simulink model "SOCPIControlBenchmarkRealVarLParGH"  (R2019b)
settings: Solver=FixedStepAuto  StartTime=0.0  StopTime=50000  FixedStep=0.01  RelTol=1e-3
values from neighbouring files (symbols this model uses):
  kio = 0.6    [benchmarkPIDStartRealVarLParGH.m]
  kpo = 0.11    [benchmarkPIDStartRealVarLParGH.m]
  maxKi = 0.3    [benchmarkPIDStartRealVarLParGH.m]
  maxKp = 0.3    [benchmarkPIDStartRealVarLParGH.m]
  minKi = 0.01    [benchmarkPIDStartRealVarLParGH.m]
  minKp = 0.01    [benchmarkPIDStartRealVarLParGH.m]
  N = 100    [benchmarkPIDStartRealVarLParGH.m]
  optimPeriod = 300    [benchmarkPIDStartRealVarLParGH.m]
  OVLim = 5    [benchmarkPIDStartRealVarLParGH.m]
  refAmplitude = 50    [benchmarkPIDStartRealVarLParGH.m]
  refSignalPeriod = optimPeriod    (= 300)    [benchmarkPIDStartRealVarLParGH.m]
  resetThreshold = 0.1    [benchmarkPIDStartRealVarLParGH.m]
undefined symbols (not defined in the file or in its folder): sigbuilder_block
libraries: dspmathops x3, simulink x3
(part 1 of 2)
settings Model: Creator=jairo  LastModifiedBy=jairo
settings DataIOCC: ReturnWorkspaceOutputs=off

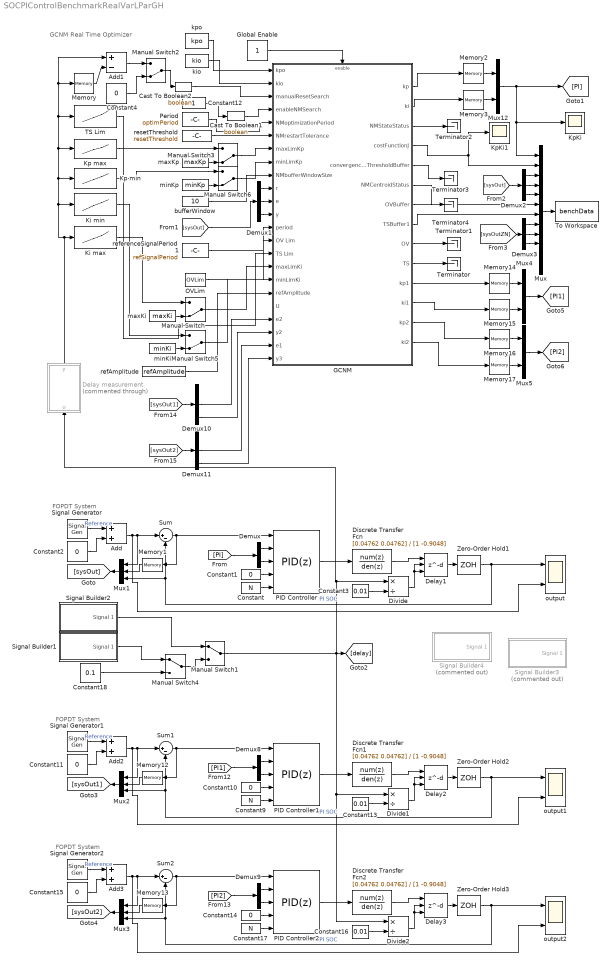
== system SOCPIControlBenchmarkRealVarLParGH ==
  note: FOPDT System
  note: GCNM Real Time Optimizer
  note: FOPDT System
  note: FOPDT System
  Add : Sum
  Add1 : Sum  Inputs=+-
  Add2 : Sum
  Add3 : Sum
  Cast To Boolean1 : DataTypeConversion  OutDataTypeStr=boolean
  Cast To Boolean2 : DataTypeConversion  OutDataTypeStr=boolean
  Constant : Constant  Value=N
  Constant{1..2,4,10..11,14..15} (7 alike) : Constant  Value=0
  Constant12 : Constant  OutDataTypeStr=boolean
  Constant13 : Constant  Value=0.01
  Constant16 : Constant  Value=0.01
  Constant17 : Constant  Value=N
  Constant18 : Constant  Value=0.1
  Constant3 : Constant  Value=0.01
  Constant9 : Constant  Value=N
  Delay measurement : MATLAB Function  Commented=through  TreatAsAtomicUnit=on
  Delay1 : Delay  DelayLengthSource=Input port  DelayLengthUpperLimit=1000  InitialConditionSource=Input port
      settings: InputPortMap=u0,p1,p4
  Delay2 : Delay  DelayLengthSource=Input port  DelayLengthUpperLimit=1000  InitialConditionSource=Input port
      settings: InputPortMap=u0,p1,p4
  Delay3 : Delay  DelayLengthSource=Input port  DelayLengthUpperLimit=1000  InitialConditionSource=Input port
      settings: InputPortMap=u0,p1,p4
  Demux : Demux  Outputs=2
  Demux{1..3,10..11} (5 alike) : Demux  Outputs=3
  Demux8 : Demux  Outputs=2
  Demux9 : Demux  Outputs=2
  Discrete Transfer Fcn : DiscreteTransferFcn  Numerator=[0.04762 0.04762]  Denominator=[1 -0.9048]
  Discrete Transfer Fcn1 : DiscreteTransferFcn  Numerator=[0.04762 0.04762]  Denominator=[1 -0.9048]
  Discrete Transfer Fcn2 : DiscreteTransferFcn  Numerator=[0.04762 0.04762]  Denominator=[1 -0.9048]
  Divide : Product  Inputs=*/
  Divide1 : Product  Inputs=*/
  Divide2 : Product  Inputs=*/
  GCNM : Subsystem
  Global Enable : Constant
  Ki max : Lookup_n-D  NumberOfTableDimensions=1  BreakpointsForDimension1=[0.1 0.5 1 2 3 4 5 6 7 8 9 10]  UseOneInputPortForAllInputData=on  Table=|  InternalRulePriority=Speed  RndMeth=Simplest  InputSameDT=on
      | [3
      | 1.61
      | 0.9
      | 0.4
      | 0.4
      | 0.3
      | 0.18
      | 0.15
      | 0.12
      | 0.1
      | 0.09
      | 0.07]
  Ki min : Lookup_n-D  NumberOfTableDimensions=1  BreakpointsForDimension1=[0.1 0.5 1 2 3 4 5 6 7 8 9 10]  UseOneInputPortForAllInputData=on  Table=|  InternalRulePriority=Speed  RndMeth=Simplest  InputSameDT=on
      | [0.8
      | 0.41
      | 0.21
      | 0.21
      | 0.11
      | 0.11
      | 0.061
      | 0.06
      | 0.061
      | 0.061
      | 0.061
      | 0.041]
  Kp max : Lookup_n-D  NumberOfTableDimensions=1  BreakpointsForDimension1=[0.1 0.5 1 2 3 4 5 6 7 8 9 10]  UseOneInputPortForAllInputData=on  Table=|  InternalRulePriority=Speed  RndMeth=Simplest  InputSameDT=on
      | [3
      | 2.21
      | 1.8
      | 1.1
      | 1
      | 0.9
      | 0.68
      | 0.73
      | 0.69
      | 0.67
      | 0.63
      | 0.54]
  Kp min : Lookup_n-D  NumberOfTableDimensions=1  BreakpointsForDimension1=[0.1 0.5 1 2 3 4 5 6 7 8 9 10]  UseOneInputPortForAllInputData=on  Table=|  InternalRulePriority=Speed  RndMeth=Simplest  InputSameDT=on
      | [0.1
      | 0.01
      | 0.01
      | 0.01
      | 0.01
      | 0.01
      | 0.01
      | 0.01
      | 0.01
      | 0.01
      | 0.01
      | 0.01
      | ]
  KpKi : Scope
  KpKi1 : Scope
  Manual Switch{,2..3,5..6} (5 alike) : ManualSwitch  CurrentSetting=0
  Manual Switch1 : ManualSwitch
  Manual Switch4 : ManualSwitch
  Memory{,1,12..13} (4 alike) : Memory
  Memory{14..17} (4 alike) : Memory  InitialCondition=0.1
  Memory2 : Memory  InitialCondition=kpo
  Memory3 : Memory  InitialCondition=kio
  Mux : Mux  Inputs=12
  Mux1 : Mux  Inputs=3
  Mux12 : Mux  Inputs=2
  Mux2 : Mux  Inputs=3
  Mux3 : Mux  Inputs=3
  Mux4 : Mux  Inputs=2
  Mux5 : Mux  Inputs=2
  OVLim : Constant  Value=OVLim
  PID Controller : simulink/Continuous/PID Controller  Controller=PID  Form=Parallel  TimeDomain=Discrete-time  SampleTime=0.1  IntegratorMethod=Forward Euler  FilterMethod=Forward Euler  ControllerParametersSource=external  P=1  I=100  D=0  UseFilter=on  N=100  TunerSelectOption=Transfer Function Based (PID Tuner App)  InitialConditionSource=internal  InitialConditionForIntegrator=0  InitialConditionForFilter=0  DifferentiatorICPrevScaledInput=0  ExternalReset=none  TrackingMode=off  Kt=1  LimitOutput=off  UpperSaturationLimit=inf  LowerSaturationLimit=-inf  LinearizeAsGain=on  AntiWindupMode=none  Kb=1  POutMin=[]  POutMax=[]  IOutMin=[]  IOutMax=[]  DOutMin=[]  DOutMax=[]  NOutMin=[]  NOutMax=[]  SumOutMin=[]  SumOutMax=[]  SaturationOutMin=[]  SaturationOutMax=[]  PParamMin=[]  PParamMax=[]  IParamMin=[]  IParamMax=[]  DParamMin=[]  DParamMax=[]  NParamMin=[]  NParamMax=[]  KbParamMin=[]  KbParamMax=[]  KtParamMin=[]  KtParamMax=[]  KbOutMin=[]  KbOutMax=[]  KtOutMin=[]  KtOutMax=[]  IntegratorOutMin=[]  IntegratorOutMax=[]  FilterOutMin=[]  FilterOutMax=[]  SumI1OutMin=[]  SumI1OutMax=[]  SumI2OutMin=[]  SumI2OutMax=[]  SumI3OutMin=[]  SumI3OutMax=[]  SumI4OutMin=[]  SumI4OutMax=[]  SumDOutMin=[]  SumDOutMax=[]  DifferentiatorOutMin=[]  DifferentiatorOutMax=[]  FilterDiffOutCoefMin=[]  FilterDiffOutCoefMax=[]  ReciprocalOutMin=[]  ReciprocalOutMax=[]  SumDenOutMin=[]  SumDenOutMax=[]  SumNumOutMin=[]  SumNumOutMax=[]  DivideOutMin=[]  DivideOutMax=[]  IntegratorContinuousStateAttributes=''  IntegratorStateMustResolveToSignalObject=off  IntegratorRTWStateStorageClass=Auto  FilterContinuousStateAttributes=''  FilterStateMustResolveToSignalObject=off  FilterRTWStateStorageClass=Auto  ParallelPVariant=ExternalParameters  IdealPVariant=Disabled  IVariant=ExternalParameters  DVariant=ExternalParameters  IntegratorVariant=Discrete  SatVariant=Disabled  AWVariant=Passthrough  PCopyVariant=Disabled  TRVariant=Disabled  FdbkBlocksVariant=Forward  IdealPFdbkVariant=Disabled  SatFdbkVariant=Disabled  DerivativeFilterVariant=ForwardEulerFilter  NVariant=ExternalParameters  NCopyVariant=Disabled  FilterICVariant=InternalICsFilter  IntegratorICVariant=InternalICs  ExternalResetVariant=Disabled  TRSumVariant=Passthrough  SumFdbkVariant=Disabled  SumVariant=Sum_PID
  PID Controller1 : simulink/Continuous/PID Controller  Controller=PID  Form=Parallel  TimeDomain=Discrete-time  SampleTime=0.1  IntegratorMethod=Forward Euler  FilterMethod=Forward Euler  ControllerParametersSource=external  P=1  I=100  D=0  UseFilter=on  N=100  TunerSelectOption=Transfer Function Based (PID Tuner App)  InitialConditionSource=internal  InitialConditionForIntegrator=0  InitialConditionForFilter=0  DifferentiatorICPrevScaledInput=0  ExternalReset=none  TrackingMode=off  Kt=1  LimitOutput=off  UpperSaturationLimit=inf  LowerSaturationLimit=-inf  LinearizeAsGain=on  AntiWindupMode=none  Kb=1  POutMin=[]  POutMax=[]  IOutMin=[]  IOutMax=[]  DOutMin=[]  DOutMax=[]  NOutMin=[]  NOutMax=[]  SumOutMin=[]  SumOutMax=[]  SaturationOutMin=[]  SaturationOutMax=[]  PParamMin=[]  PParamMax=[]  IParamMin=[]  IParamMax=[]  DParamMin=[]  DParamMax=[]  NParamMin=[]  NParamMax=[]  KbParamMin=[]  KbParamMax=[]  KtParamMin=[]  KtParamMax=[]  KbOutMin=[]  KbOutMax=[]  KtOutMin=[]  KtOutMax=[]  IntegratorOutMin=[]  IntegratorOutMax=[]  FilterOutMin=[]  FilterOutMax=[]  SumI1OutMin=[]  SumI1OutMax=[]  SumI2OutMin=[]  SumI2OutMax=[]  SumI3OutMin=[]  SumI3OutMax=[]  SumI4OutMin=[]  SumI4OutMax=[]  SumDOutMin=[]  SumDOutMax=[]  DifferentiatorOutMin=[]  DifferentiatorOutMax=[]  FilterDiffOutCoefMin=[]  FilterDiffOutCoefMax=[]  ReciprocalOutMin=[]  ReciprocalOutMax=[]  SumDenOutMin=[]  SumDenOutMax=[]  SumNumOutMin=[]  SumNumOutMax=[]  DivideOutMin=[]  DivideOutMax=[]  IntegratorContinuousStateAttributes=''  IntegratorStateMustResolveToSignalObject=off  IntegratorRTWStateStorageClass=Auto  FilterContinuousStateAttributes=''  FilterStateMustResolveToSignalObject=off  FilterRTWStateStorageClass=Auto  ParallelPVariant=ExternalParameters  IdealPVariant=Disabled  IVariant=ExternalParameters  DVariant=ExternalParameters  IntegratorVariant=Discrete  SatVariant=Disabled  AWVariant=Passthrough  PCopyVariant=Disabled  TRVariant=Disabled  FdbkBlocksVariant=Forward  IdealPFdbkVariant=Disabled  SatFdbkVariant=Disabled  DerivativeFilterVariant=ForwardEulerFilter  NVariant=ExternalParameters  NCopyVariant=Disabled  FilterICVariant=InternalICsFilter  IntegratorICVariant=InternalICs  ExternalResetVariant=Disabled  TRSumVariant=Passthrough  SumFdbkVariant=Disabled  SumVariant=Sum_PID
  PID Controller2 : simulink/Continuous/PID Controller  Controller=PID  Form=Parallel  TimeDomain=Discrete-time  SampleTime=0.1  IntegratorMethod=Forward Euler  FilterMethod=Forward Euler  ControllerParametersSource=external  P=1  I=100  D=0  UseFilter=on  N=100  TunerSelectOption=Transfer Function Based (PID Tuner App)  InitialConditionSource=internal  InitialConditionForIntegrator=0  InitialConditionForFilter=0  DifferentiatorICPrevScaledInput=0  ExternalReset=none  TrackingMode=off  Kt=1  LimitOutput=off  UpperSaturationLimit=inf  LowerSaturationLimit=-inf  LinearizeAsGain=on  AntiWindupMode=none  Kb=1  POutMin=[]  POutMax=[]  IOutMin=[]  IOutMax=[]  DOutMin=[]  DOutMax=[]  NOutMin=[]  NOutMax=[]  SumOutMin=[]  SumOutMax=[]  SaturationOutMin=[]  SaturationOutMax=[]  PParamMin=[]  PParamMax=[]  IParamMin=[]  IParamMax=[]  DParamMin=[]  DParamMax=[]  NParamMin=[]  NParamMax=[]  KbParamMin=[]  KbParamMax=[]  KtParamMin=[]  KtParamMax=[]  KbOutMin=[]  KbOutMax=[]  KtOutMin=[]  KtOutMax=[]  IntegratorOutMin=[]  IntegratorOutMax=[]  FilterOutMin=[]  FilterOutMax=[]  SumI1OutMin=[]  SumI1OutMax=[]  SumI2OutMin=[]  SumI2OutMax=[]  SumI3OutMin=[]  SumI3OutMax=[]  SumI4OutMin=[]  SumI4OutMax=[]  SumDOutMin=[]  SumDOutMax=[]  DifferentiatorOutMin=[]  DifferentiatorOutMax=[]  FilterDiffOutCoefMin=[]  FilterDiffOutCoefMax=[]  ReciprocalOutMin=[]  ReciprocalOutMax=[]  SumDenOutMin=[]  SumDenOutMax=[]  SumNumOutMin=[]  SumNumOutMax=[]  DivideOutMin=[]  DivideOutMax=[]  IntegratorContinuousStateAttributes=''  IntegratorStateMustResolveToSignalObject=off  IntegratorRTWStateStorageClass=Auto  FilterContinuousStateAttributes=''  FilterStateMustResolveToSignalObject=off  FilterRTWStateStorageClass=Auto  ParallelPVariant=ExternalParameters  IdealPVariant=Disabled  IVariant=ExternalParameters  DVariant=ExternalParameters  IntegratorVariant=Discrete  SatVariant=Disabled  AWVariant=Passthrough  PCopyVariant=Disabled  TRVariant=Disabled  FdbkBlocksVariant=Forward  IdealPFdbkVariant=Disabled  SatFdbkVariant=Disabled  DerivativeFilterVariant=ForwardEulerFilter  NVariant=ExternalParameters  NCopyVariant=Disabled  FilterICVariant=InternalICsFilter  IntegratorICVariant=InternalICs  ExternalResetVariant=Disabled  TRSumVariant=Passthrough  SumFdbkVariant=Disabled  SumVariant=Sum_PID
  Period : Constant  Value=optimPeriod  OutDataTypeStr=double
  Signal Generator : SignalGenerator  WaveForm=square  Frequency=1/refSignalPeriod
  Signal Generator1 : SignalGenerator  WaveForm=square  Frequency=1/refSignalPeriod
  Signal Generator2 : SignalGenerator  WaveForm=square  Frequency=1/refSignalPeriod
  Signal Builder1 : Subsystem  Tag=STV Subsys  LoadFcn=sigbuilder_block('load');  StartFcn=sigbuilder_block('start');  StopFcn=sigbuilder_block('stop');  ClipboardFcn=sigbuilder_block('clipboard');  mask(Sigbuilder block){tuvar=[0:10]}
      mask help: Simulink:masks:SigbuilderBlock_MD
      mask init:
      | if ~strcmp(get_param(bdroot(gcbh),'SimulationStatus'),'stopped') tuvar = sigbuilder_block('maskInit'); end
      settings: CopyFcn=sigbuilder_block('copy');  DeleteFcn=sigbuilder_block('delete');  ModelCloseFcn=sigbuilder_block('modelClose');  PreSaveFcn=sigbuilder_block('preSave');  PauseFcn=sigbuilder_block('pause');  ContinueFcn=sigbuilder_block('continue');  NameChangeFcn=sigbuilder_block('namechange');  OpenFcn=sigbuilder_block('open',[5.4 30.6 1141.2 522.6 ]);  CloseFcn=sigbuilder_block('close');
      mask Display: plot(0, 0, 100, 100,[2, 2, 32, 32, 2], [68, 8, 8, 68, 68],[32, 2], [38, 38], [32, 19, 2],[53, 60, 44], [32, 17, 17, 2],[16, 16, 31, 31]);txt = getActiveGroup(gcbh);text(2, 100, txt,'verticalAlignment', 'top');
  Signal Builder2 : Subsystem  Tag=STV Subsys  LoadFcn=sigbuilder_block('load',[0.75 38.25 1141.5 514.5 ]);  StartFcn=sigbuilder_block('start');  StopFcn=sigbuilder_block('stop');  ClipboardFcn=sigbuilder_block('clipboard');  mask(Sigbuilder block){tuvar=[0:10]}
      mask help: Simulink:masks:SigbuilderBlock_MD
      mask init:
      | if ~strcmp(get_param(bdroot(gcbh),'SimulationStatus'),'stopped') tuvar = sigbuilder_block('maskInit'); end
      settings: CopyFcn=sigbuilder_block('copy');  DeleteFcn=sigbuilder_block('delete');  ModelCloseFcn=sigbuilder_block('modelClose');  PreSaveFcn=sigbuilder_block('preSave');  PauseFcn=sigbuilder_block('pause');  ContinueFcn=sigbuilder_block('continue');  NameChangeFcn=sigbuilder_block('namechange');  OpenFcn=sigbuilder_block('open',[0.75 38.25 1141.5 514.5 ]);  CloseFcn=sigbuilder_block('close');
      mask Display: plot(0, 0, 100, 100,[2, 2, 32, 32, 2], [68, 8, 8, 68, 68],[32, 2], [38, 38], [32, 19, 2],[53, 60, 44], [32, 17, 17, 2],[16, 16, 31, 31]);txt = getActiveGroup(gcbh);text(2, 100, txt,'verticalAlignment', 'top');
  Signal Builder3 : Subsystem  Tag=STV Subsys  Commented=on  LoadFcn=sigbuilder_block('load');  StartFcn=sigbuilder_block('start');  StopFcn=sigbuilder_block('stop');  ClipboardFcn=sigbuilder_block('clipboard');  mask(Sigbuilder block){tuvar=[0:10]}
      mask help: Simulink:masks:SigbuilderBlock_MD
      mask init:
      | if ~strcmp(get_param(bdroot(gcbh),'SimulationStatus'),'stopped') tuvar = sigbuilder_block('maskInit'); end
      settings: CopyFcn=sigbuilder_block('copy');  DeleteFcn=sigbuilder_block('delete');  ModelCloseFcn=sigbuilder_block('modelClose');  PreSaveFcn=sigbuilder_block('preSave');  PauseFcn=sigbuilder_block('pause');  ContinueFcn=sigbuilder_block('continue');  NameChangeFcn=sigbuilder_block('namechange');  OpenFcn=sigbuilder_block('open',[5.4 33 1141.2 514.8 ]);  CloseFcn=sigbuilder_block('close');
      mask Display: plot(0, 0, 100, 100,[2, 2, 32, 32, 2], [68, 8, 8, 68, 68],[32, 2], [38, 38], [32, 19, 2],[53, 60, 44], [32, 17, 17, 2],[16, 16, 31, 31]);txt = getActiveGroup(gcbh);text(2, 100, txt,'verticalAlignment', 'top');
  Signal Builder4 : Subsystem  Tag=STV Subsys  Commented=on  LoadFcn=sigbuilder_block('load');  StartFcn=sigbuilder_block('start');  StopFcn=sigbuilder_block('stop');  ClipboardFcn=sigbuilder_block('clipboard');  mask(Sigbuilder block){tuvar=[0:10]}
      mask help: Simulink:masks:SigbuilderBlock_MD
      mask init:
      | if ~strcmp(get_param(bdroot(gcbh),'SimulationStatus'),'stopped') tuvar = sigbuilder_block('maskInit'); end
      settings: CopyFcn=sigbuilder_block('copy');  DeleteFcn=sigbuilder_block('delete');  ModelCloseFcn=sigbuilder_block('modelClose');  PreSaveFcn=sigbuilder_block('preSave');  PauseFcn=sigbuilder_block('pause');  ContinueFcn=sigbuilder_block('continue');  NameChangeFcn=sigbuilder_block('namechange');  OpenFcn=sigbuilder_block('open',[5.4 30.6 1141.2 522.6 ]);  CloseFcn=sigbuilder_block('close');
      mask Display: plot(0, 0, 100, 100,[2, 2, 32, 32, 2], [68, 8, 8, 68, 68],[32, 2], [38, 38], [32, 19, 2],[53, 60, 44], [32, 17, 17, 2],[16, 16, 31, 31]);txt = getActiveGroup(gcbh);text(2, 100, txt,'verticalAlignment', 'top');
  Sum : Sum  Inputs=|+-
  Sum1 : Sum  Inputs=|+-
  Sum2 : Sum  Inputs=|+-
  TS Lim : Lookup_n-D  NumberOfTableDimensions=1  BreakpointsForDimension1=[0.1 0.5 1 2 3 4 5 6 7 8 9 10]  UseOneInputPortForAllInputData=on  Table=|  InternalRulePriority=Speed  RndMeth=Simplest  InputSameDT=on
      | [100
      | 100
      | 100
      | 100
      | 100
      | 100
      | 100
      | 100
      | 100
      | 100
      | 100
      | 100]
  Terminator{,1..4} (5 alike) : Terminator
  To Workspace : ToWorkspace  VariableName=benchData  SaveFormat=Timeseries  SampleTime=-1
  Zero-Order Hold1 : ZeroOrderHold  SampleTime=-1
  Zero-Order Hold2 : ZeroOrderHold  SampleTime=-1
  Zero-Order Hold3 : ZeroOrderHold  SampleTime=-1
  bufferWindow : Constant  Value=10  OutDataTypeStr=uint16
  kio : Constant  Value=kio  OutDataTypeStr=double
  kpo : Constant  Value=kpo  OutDataTypeStr=double
  maxKi : Constant  Value=maxKi  VectorParams1D=off  OutDataTypeStr=double
  maxKp : Constant  Value=maxKp  OutDataTypeStr=double
  minKi : Constant  Value=minKi  OutDataTypeStr=double
  minKp : Constant  Value=minKp  OutDataTypeStr=double
  output : Scope  NumInputPorts=2
  output1 : Scope  NumInputPorts=2
  output2 : Scope  NumInputPorts=2
  refAmplitude : Constant  Value=refAmplitude  OutDataTypeStr=double
  referenceSignalPeriod1 : Constant  Value=refSignalPeriod
  resetThreshold : Constant  Value=resetThreshold
  wires:
  PID Controller/1 -> Discrete Transfer Fcn/1
  Sum/1 -> Memory1/1, PID Controller/1
  resetThreshold/1 -> GCNM/6(NMrestartTolerance)
  bufferWindow/1 -> GCNM/9(NMbufferWindowSize)
  Cast To Boolean1/1 -> GCNM/4(enableNMSearch)
  kio/1 -> GCNM/2(kio)
  Constant12/1 -> Cast To Boolean1/1
  Global Enable/1 -> GCNM/Enable
  kpo/1 -> GCNM/1(kpo)
  Period/1 -> GCNM/5(NMoptimizationPeriod)
  GCNM/4(costFunctionJ) -> Mux/2, KpKi1/1
  OVLim/1 -> GCNM/14("  OV Lim")
  Zero-Order Hold1/1 -> Sum/2, Mux1/3, output/1  "PI SOC"
  GCNM/1("  kp") -> Memory2/1
  GCNM/2("  ki") -> Memory3/1
  Mux/1 -> To Workspace/1
  Constant/1 -> PID Controller/5
  Constant1/1 -> PID Controller/4
  Demux/1 -> PID Controller/2
  Demux/2 -> PID Controller/3
  Mux1/1 -> [sysOut]
  [sysOut] -> Demux1/1
  Demux1/1 -> GCNM/10(r)
  Demux1/2 -> GCNM/11("  e")
  Demux1/3 -> GCNM/12("  y")
  [sysOut] -> Demux2/1
  Demux2/1 -> Mux/3
  Demux2/2 -> Mux/4
  Demux2/3 -> Mux/5
  [sysOutZN] -> Demux3/1
  Demux3/1 -> Mux/8
  Demux3/2 -> Mux/9
  Demux3/3 -> Mux/10
  GCNM/10(TS) -> Terminator/1
  GCNM/9(OV) -> Terminator1/1
  GCNM/8(TSBuffer1) -> Mux/7
  GCNM/7(OVBuffer) -> Mux/6
  GCNM/3(NMStateStatus) -> Terminator2/1
  GCNM/5(convergenceThresholdBuffer) -> Terminator3/1
  GCNM/6(NMCentroidStatus) -> Terminator4/1
  Signal Generator/1 -> Add/1  "Reference"
  Constant2/1 -> Add/2
  Add/1 -> Mux1/1, Sum/1, output/2
  refAmplitude/1 -> GCNM/18(refAmplitude)
  [PI] -> Demux/1
  maxKi/1 -> Manual Switch/2
  Manual Switch/1 -> GCNM/16(maxLimKi)
  Manual Switch3/1 -> GCNM/7(maxLimKp)
  maxKp/1 -> Manual Switch3/2
  Constant18/1 -> Manual Switch4/2
  Manual Switch4/1 -> Manual Switch1/2
  minKi/1 -> Manual Switch5/2
  minKp/1 -> Manual Switch6/2
  Manual Switch6/1 -> GCNM/8(minLimKp)
  Manual Switch5/1 -> GCNM/17(minLimKi)
  Divide/1 -> Delay1/3, Delay1/2
  Constant3/1 -> Divide/2
  Discrete Transfer Fcn/1 -> Delay1/1
  Delay1/1 -> Zero-Order Hold1/1
  Mux12/1 -> KpKi/1, Mux/1, [PI]
  Memory1/1 -> Mux1/2
  Memory2/1 -> Mux12/1
  Memory3/1 -> Mux12/2
  Kp max/1 -> Manual Switch3/1
  Kp min/1 -> Manual Switch6/1
  Ki max/1 -> Manual Switch/1
  Ki min/1 -> Manual Switch5/1
  TS Lim/1 -> GCNM/15(TS Lim)
  referenceSignalPeriod1/1 -> GCNM/13("  period")
  Manual Switch1/1 -> Divide2/1, Divide1/1, [delay], Delay measurement/1(u), Divide/1
  Memory/1 -> Add1/2
  Cast To Boolean2/1 -> GCNM/3(manualResetSearch)
  Signal Builder2/1(Signal 1) -> Manual Switch1/1
  Signal Builder1/1(Signal 1) -> Manual Switch4/1
  Delay measurement/1(y) -> Add1/1, Memory/1, TS Lim/1, Kp max/1, Kp min/1, Ki min/1, Ki max/1
  Add1/1 -> Manual Switch2/1
  Manual Switch2/1 -> Cast To Boolean2/1
  Constant4/1 -> Manual Switch2/2
  Constant9/1 -> PID Controller1/5
  Add2/1 -> Mux2/1, Sum1/1, output1/2
  [PI1] -> Demux8/1
  Delay2/1 -> Zero-Order Hold2/1
  Divide1/1 -> Delay2/3, Delay2/2
  PID Controller1/1 -> Discrete Transfer Fcn1/1
  Mux2/1 -> [sysOut1]
  Signal Generator1/1 -> Add2/1  "Reference"
  Constant10/1 -> PID Controller1/4
  Zero-Order Hold2/1 -> Sum1/2, Mux2/3, output1/1  "PI SOC"
  Sum1/1 -> Memory12/1, PID Controller1/1
  Demux8/1 -> PID Controller1/2
  Memory12/1 -> Mux2/2
  Demux8/2 -> PID Controller1/3
  Constant13/1 -> Divide1/2
  Discrete Transfer Fcn1/1 -> Delay2/1
  Constant11/1 -> Add2/2
  Constant15/1 -> Add3/2
  Discrete Transfer Fcn2/1 -> Delay3/1
  Constant16/1 -> Divide2/2
  Memory13/1 -> Mux3/2
  Zero-Order Hold3/1 -> Sum2/2, Mux3/3, output2/1  "PI SOC"
  Demux9/1 -> PID Controller2/2
  Divide2/1 -> Delay3/3, Delay3/2
  PID Controller2/1 -> Discrete Transfer Fcn2/1
  Constant14/1 -> PID Controller2/4
  Delay3/1 -> Zero-Order Hold3/1
  Signal Generator2/1 -> Add3/1  "Reference"
  Constant17/1 -> PID Controller2/5
  Mux3/1 -> [sysOut2]
  Sum2/1 -> Memory13/1, PID Controller2/1
  Add3/1 -> Mux3/1, Sum2/1, output2/2
  Demux9/2 -> PID Controller2/3
  [PI2] -> Demux9/1
  [sysOut1] -> Demux10/1
  [sysOut2] -> Demux11/1
  Demux10/2 -> GCNM/20("  e2")
  Demux10/3 -> GCNM/21("  y2")
  Demux11/2 -> GCNM/22("  e1")
  Demux11/3 -> GCNM/23("  y3")
  Mux4/1 -> [PI1]
  Memory15/1 -> Mux4/2
  Memory14/1 -> Mux4/1
  GCNM/11("  kp1") -> Memory14/1
  GCNM/12("  ki1") -> Memory15/1
  Mux5/1 -> [PI2]
  GCNM/14("  ki2") -> Memory17/1
  Memory17/1 -> Mux5/2
  Memory16/1 -> Mux5/1
  GCNM/13("  kp2") -> Memory16/1

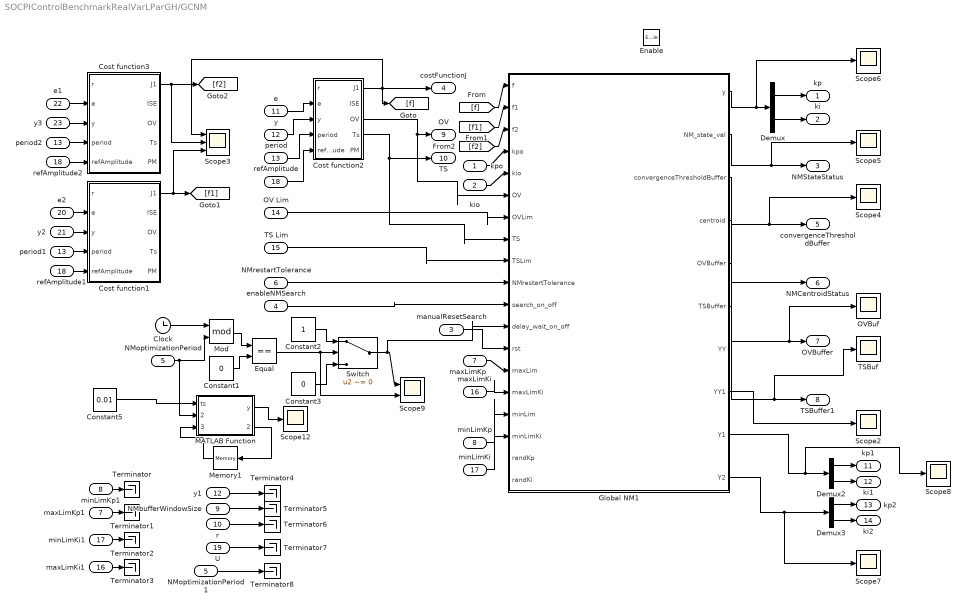
== system SOCPIControlBenchmarkRealVarLParGH/GCNM ==
  kpo : Inport  OutDataTypeStr=double
  kio : Inport  Port=2  OutDataTypeStr=double
  manualResetSearch : Inport  Port=3  OutDataTypeStr=boolean
  enableNMSearch : Inport  Port=4  OutDataTypeStr=boolean
  NMoptimizationPeriod : Inport  Port=5  OutDataTypeStr=double
  NMrestartTolerance : Inport  Port=6
  maxLimKp : Inport  Port=7  OutDataTypeStr=double
  minLimKp : Inport  Port=8  OutDataTypeStr=double
  NMbufferWindowSize : Inport  Port=9  OutDataTypeStr=uint16
  r : Inport  Port=10
  "  e" : Inport  Port=11  OutDataTypeStr=double
  "  y" : Inport  Port=12  OutDataTypeStr=double
  "  period" : Inport  Port=13  OutDataTypeStr=double
  "  OV Lim" : Inport  Port=14  OutDataTypeStr=double
  TS Lim : Inport  Port=15  OutDataTypeStr=double
  maxLimKi : Inport  Port=16  OutDataTypeStr=double
  minLimKi : Inport  Port=17  OutDataTypeStr=double
  refAmplitude : Inport  Port=18  OutDataTypeStr=double
  "  U" : Inport  Port=19  OutDataTypeStr=double
  "  e2" : Inport  Port=20  OutDataTypeStr=double
  "  y2" : Inport  Port=21  OutDataTypeStr=double
  "  e1" : Inport  Port=22  OutDataTypeStr=double
  "  y3" : Inport  Port=23  OutDataTypeStr=double
  Enable : EnablePort
  "  period1" : InportShadow  Port=13  OutDataTypeStr=double
  "  period2" : InportShadow  Port=13  OutDataTypeStr=double
  "  y1" : InportShadow  Port=12  OutDataTypeStr=double
  Clock : Clock
      settings: Decimation=1000
  Constant1 : Constant  Value=0
  Constant2 : Constant
  Constant3 : Constant  Value=0
  Constant5 : Constant  Value=0.01
  Cost function1 : Subsystem
  Cost function2 : Subsystem
  Cost function3 : Subsystem
  Demux : Demux  Outputs=2
  Demux2 : Demux  Outputs=2
  Demux3 : Demux  Outputs=2
  Equal : RelationalOperator  Operator===  RndMeth=Simplest
  Global NM1 : MATLAB Function  TreatAsAtomicUnit=on
  MATLAB Function : MATLAB Function  TreatAsAtomicUnit=on
  Memory1 : Memory  InitialCondition=300/0.01
  Mod : Math  Operator=mod  SignedPower=off  SaturateOnIntegerOverflow=on
  NMoptimizationPeriod1 : InportShadow  Port=5  OutDataTypeStr=double
  OVBuf : Scope
  Scope{2,4..8,12} (7 alike) : Scope
  Scope3 : Scope  NumInputPorts=3
  Scope9 : Scope  NumInputPorts=2
  Switch : Switch  Criteria=u2 ~= 0
  TSBuf : Scope
  Terminator{,1..8} (9 alike) : Terminator
  maxLimKi1 : InportShadow  Port=16  OutDataTypeStr=double
  maxLimKp1 : InportShadow  Port=7  OutDataTypeStr=double
  minLimKi1 : InportShadow  Port=17  OutDataTypeStr=double
  minLimKp1 : InportShadow  Port=8  OutDataTypeStr=double
  refAmplitude1 : InportShadow  Port=18  OutDataTypeStr=double
  refAmplitude2 : InportShadow  Port=18  OutDataTypeStr=double
  "  kp" : Outport  OutDataTypeStr=double
  "  ki" : Outport  Port=2  OutDataTypeStr=double
  NMStateStatus : Outport  Port=3  OutDataTypeStr=double
  costFunctionJ : Outport  Port=4  OutDataTypeStr=double
  convergenceThresholdBuffer : Outport  Port=5  OutDataTypeStr=double
  NMCentroidStatus : Outport  Port=6  OutDataTypeStr=double
  OVBuffer : Outport  Port=7  OutDataTypeStr=double
  TSBuffer1 : Outport  Port=8  OutDataTypeStr=double
  OV : Outport  Port=9  OutDataTypeStr=double
  TS : Outport  Port=10  OutDataTypeStr=double
  "  kp1" : Outport  Port=11  OutDataTypeStr=double
  "  ki1" : Outport  Port=12  OutDataTypeStr=double
  "  kp2" : Outport  Port=13  OutDataTypeStr=double
  "  ki2" : Outport  Port=14  OutDataTypeStr=double
  wires:
  Demux/2 -> "  ki"/1
  Demux/1 -> "  kp"/1
  NMrestartTolerance/1 -> Global NM1/10(NMrestartTolerance)
  manualResetSearch/1 -> Global NM1/13(rst)
  enableNMSearch/1 -> Global NM1/11(search_on_off)
  minLimKp/1 -> Global NM1/16(minLim)
  maxLimKp/1 -> Global NM1/14(maxLim)
  Global NM1/2(NM_state_val) -> Scope5/1, NMStateStatus/1
  Global NM1/3(convergenceThresholdBuffer) -> convergenceThresholdBuffer/1, Scope4/1
  Global NM1/4(centroid) -> NMCentroidStatus/1
  Global NM1/1(y) -> Scope6/1, Demux/1
  kpo/1 -> Global NM1/4(kpo)
  kio/1 -> Global NM1/5(kio)
  Cost function2/3(OV) -> OV/1, Global NM1/6(OV)
  "  y"/1 -> Cost function2/3(y)
  "  e"/1 -> Cost function2/2(e)
  Global NM1/5(OVBuffer) -> OVBuf/1, OVBuffer/1
  "  period"/1 -> Cost function2/4(period)
  "  OV Lim"/1 -> Global NM1/7(OVLim)
  Cost function2/4(Ts) -> TS/1, Global NM1/8(TS)
  TS Lim/1 -> Global NM1/9(TSLim)
  Global NM1/6(TSBuffer) -> TSBuffer1/1, TSBuf/1
  Cost function2/1(J1) -> Scope3/1, [f], costFunctionJ/1
  Clock/1 -> Mod/1
  NMoptimizationPeriod/1 -> MATLAB Function/2(NMOptimPeriod), Mod/2
  Constant1/1 -> Equal/2
  Mod/1 -> Equal/1
  Constant2/1 -> Switch/1
  Constant3/1 -> Switch/3
  maxLimKi/1 -> Global NM1/15(maxLimKi)
  minLimKi/1 -> Global NM1/17(minLimKi)
  refAmplitude/1 -> Cost function2/5(refAmplitude)
  r/1 -> Terminator6/1
  "  U"/1 -> Terminator7/1
  "  e2"/1 -> Cost function1/2(e)
  "  y2"/1 -> Cost function1/3(y)
  "  period1"/1 -> Cost function1/4(period)
  refAmplitude1/1 -> Cost function1/5(refAmplitude)
  "  e1"/1 -> Cost function3/2(e)
  "  y3"/1 -> Cost function3/3(y)
  refAmplitude2/1 -> Cost function3/5(refAmplitude)
  "  period2"/1 -> Cost function3/4(period)
  Cost function1/1(J1) -> Scope3/3, [f1]
  [f] -> Global NM1/1(f)
  [f1] -> Global NM1/2(f1)
  [f2] -> Global NM1/3(f2)
  Global NM1/8(YY1) -> Scope2/1
  Demux2/2 -> "  ki1"/1
  Demux3/2 -> "  ki2"/1
  Demux3/1 -> "  kp2"/1
  Global NM1/9(Y1) -> Scope8/1, Demux2/1
  Global NM1/10(Y2) -> Scope7/1, Demux3/1
  Demux2/1 -> "  kp1"/1
  Cost function3/1(J1) -> Scope3/2, [f2]
  Equal/1 -> Scope9/2, Switch/2
  Switch/1 -> Global NM1/12(delay_wait_on_off), Scope9/1
  MATLAB Function/2(counter1) -> Memory1/1
  Memory1/1 -> MATLAB Function/3(counter)
  Constant5/1 -> MATLAB Function/1(ts)
  MATLAB Function/1(y) -> Scope12/1
  minLimKp1/1 -> Terminator/1
  maxLimKp1/1 -> Terminator1/1
  minLimKi1/1 -> Terminator2/1
  maxLimKi1/1 -> Terminator3/1
  "  y1"/1 -> Terminator4/1
  NMbufferWindowSize/1 -> Terminator5/1
  NMoptimizationPeriod1/1 -> Terminator8/1

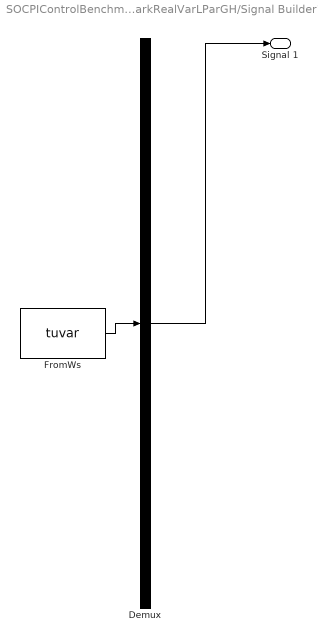
== system SOCPIControlBenchmarkRealVarLParGH/Signal Builder1 ==
  Demux : Demux  Tag=STV Demux  Outputs=1
  FromWs : FromWorkspace  Tag=STV FromWs  VariableName=tuvar  SampleTime=0
      SigBuilderData=|
      | common.afterFinalStr = 'Extrapolate'
      | common.sampleTime = 0
      | dataSet.timeRange = [0 50000]
      | dataSet.name = 'Group 1'
      | sbobj.Groups.Name = 'Group 1'
      | sbobj.Groups.Signals.Name = 'Signal 1'
      | sbobj.Groups.Signals.XData = [0 12000 21000 21000 50000]
      | sbobj.Groups.Signals.YData = [1 1 1 8 8]
      | sbobj.Groups.TimeRange = [0 50000]
  Signal 1 : Outport  Tag=STV Outport
  wires:
  FromWs/1 -> Demux/1
  Demux/1 -> Signal 1/1

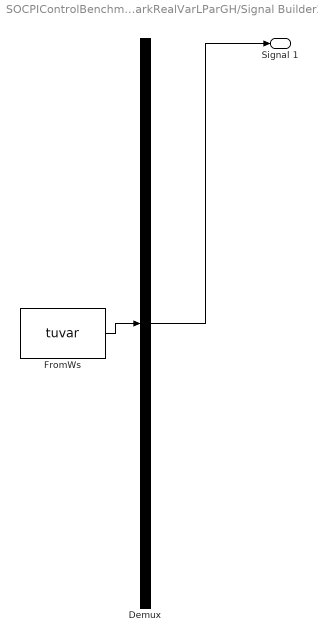
== system SOCPIControlBenchmarkRealVarLParGH/Signal Builder2 ==
  Demux : Demux  Tag=STV Demux  Outputs=1
  FromWs : FromWorkspace  Tag=STV FromWs  VariableName=tuvar  SampleTime=0
      SigBuilderData=|
      | common.afterFinalStr = 'Extrapolate'
      | common.sampleTime = 0
      | dataSet.timeRange = [0 50000]
      | dataSet.name = 'Group 1'
      | sbobj.Groups.Name = 'Group 1'
      | sbobj.Groups.Signals.Name = 'Signal 1'
      | sbobj.Groups.Signals.XData = [0 15000 15000 30000 30000 50000]
      | sbobj.Groups.Signals.YData = [0.4 0.4 1 1 10 10]
      | sbobj.Groups.TimeRange = [0 50000]
  Signal 1 : Outport  Tag=STV Outport
  wires:
  Demux/1 -> Signal 1/1
  FromWs/1 -> Demux/1

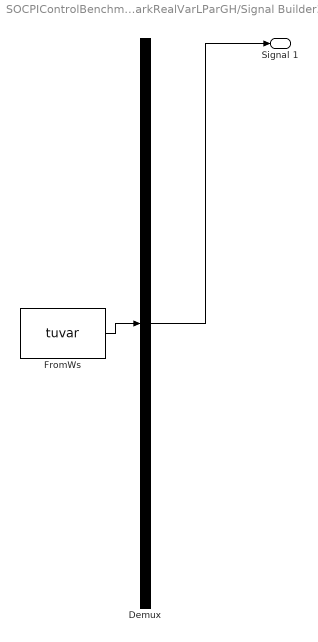
== system SOCPIControlBenchmarkRealVarLParGH/Signal Builder3 ==
  Demux : Demux  Tag=STV Demux  Outputs=1
  FromWs : FromWorkspace  Tag=STV FromWs  VariableName=tuvar  SampleTime=0
      SigBuilderData=|
      | common.afterFinalStr = 'Extrapolate'
      | common.sampleTime = 0
      | dataSet.timeRange = [0 50000]
      | dataSet.name = 'Group 1'
      | sbobj.Groups.Name = 'Group 1'
      | sbobj.Groups.Signals.Name = 'Signal 1'
      | sbobj.Groups.Signals.XData = [0 12000 12000 21000 21000 36000 36000 50000]
      | sbobj.Groups.Signals.YData = [0.1 0.1 5 5 8 8 3 3]
      | sbobj.Groups.TimeRange = [0 50000]
  Signal 1 : Outport  Tag=STV Outport
  wires:
  FromWs/1 -> Demux/1
  Demux/1 -> Signal 1/1

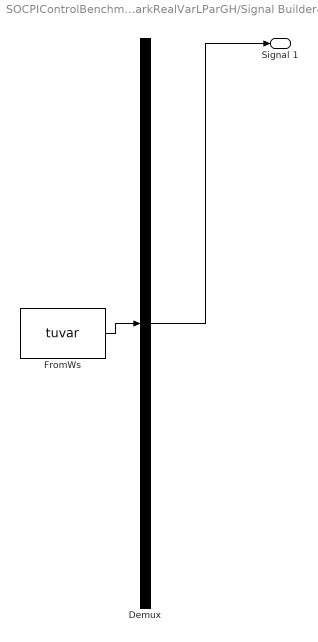
== system SOCPIControlBenchmarkRealVarLParGH/Signal Builder4 ==
  Demux : Demux  Tag=STV Demux  Outputs=1
  FromWs : FromWorkspace  Tag=STV FromWs  VariableName=tuvar  SampleTime=0
      SigBuilderData=|
      | common.afterFinalStr = 'Extrapolate'
      | common.sampleTime = 0
      | dataSet.timeRange = [0 50000]
      | dataSet.name = 'Group 1'
      | sbobj.Groups.Name = 'Group 1'
      | sbobj.Groups.Signals.Name = 'Signal 1'
      | sbobj.Groups.Signals.XData = [0 12000 12000 21000 21000 36000 36000 50000]
      | sbobj.Groups.Signals.YData = [7.98 7.98 5.86 5.86 0.64 0.64 4.2 4.2]
      | sbobj.Groups.TimeRange = [0 50000]
  Signal 1 : Outport  Tag=STV Outport
  wires:
  Demux/1 -> Signal 1/1
  FromWs/1 -> Demux/1

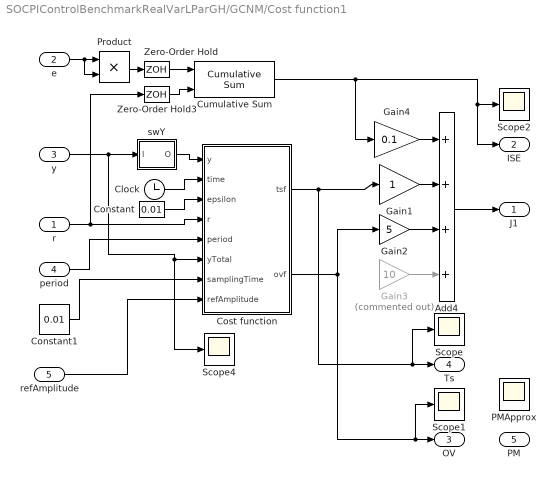
== system SOCPIControlBenchmarkRealVarLParGH/GCNM/Cost function1 ==
  r : Inport
  e : Inport  Port=2
  y : Inport  Port=3
  period : Inport  Port=4
  refAmplitude : Inport  Port=5
  Add4 : Sum  Inputs=++++
  Clock : Clock
  Constant : Constant  Value=0.01
  Constant1 : Constant  Value=0.01
  Cost function : MATLAB Function  TreatAsAtomicUnit=on
  Cumulative Sum : dspmathops/Cumulative Sum  dim=Channels (running sum)  InputProcessing=Columns as channels (frame based)  reset_popup=Falling edge  roundingMode=Floor  overflowMode=off  outputDataTypeStr=Inherit: Same as accumulator  outputMin=[]  outputMax=[]  outputLastDataTypeStr=Inherit: Same as accumulator
      settings: SourceProductName=DSP System Toolbox
  Gain1 : Gain
  Gain2 : Gain  Gain=5
  Gain3 : Gain  Commented=on  Gain=10
  Gain4 : Gain  Gain=0.1
  PMApprox : Scope
  Product : Product
  Scope{,1..2,4} (4 alike) : Scope
  Zero-Order Hold : ZeroOrderHold  SampleTime=-1
  Zero-Order Hold3 : ZeroOrderHold  SampleTime=-1
  swY : Subsystem
  J1 : Outport
  ISE : Outport  Port=2
  OV : Outport  Port=3
  Ts : Outport  Port=4
  PM : Outport  Port=5
  wires:
  Gain4/1 -> Add4/1
  Cost function/2(ovf) -> OV/1, Scope1/1, Gain2/1
  Cost function/1(tsf) -> Ts/1, Scope/1, Gain1/1
  Gain3/1 -> Add4/4
  refAmplitude/1 -> Cost function/8(refAmplitude)
  Gain1/1 -> Add4/2
  Constant1/1 -> Cost function/7(samplingTime)
  period/1 -> Cost function/5(period)
  Gain2/1 -> Add4/3
  Add4/1 -> J1/1
  y/1 -> swY/1(I), Cost function/6(yTotal), Scope4/1
  Constant/1 -> Cost function/3(epsilon)
  Product/1 -> Zero-Order Hold/1
  Clock/1 -> Cost function/2(time)
  swY/1(O) -> Cost function/1(y)
  r/1 -> Cost function/4(r), Zero-Order Hold3/1
  Zero-Order Hold/1 -> Cumulative Sum/1
  e/1 -> Product/1, Product/2
  Zero-Order Hold3/1 -> Cumulative Sum/2
  Cumulative Sum/1 -> Scope2/1, ISE/1, Gain4/1

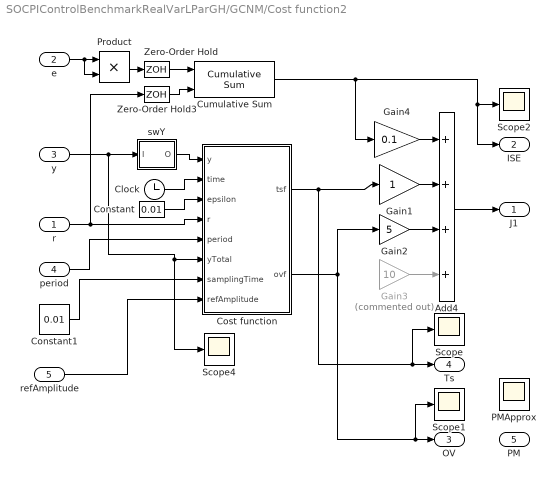
== system SOCPIControlBenchmarkRealVarLParGH/GCNM/Cost function2 ==
  r : Inport
  e : Inport  Port=2
  y : Inport  Port=3
  period : Inport  Port=4
  refAmplitude : Inport  Port=5
  Add4 : Sum  Inputs=++++
  Clock : Clock
  Constant : Constant  Value=0.01
  Constant1 : Constant  Value=0.01
  Cost function : MATLAB Function  TreatAsAtomicUnit=on
  Cumulative Sum : dspmathops/Cumulative Sum  dim=Channels (running sum)  InputProcessing=Columns as channels (frame based)  reset_popup=Falling edge  roundingMode=Floor  overflowMode=off  outputDataTypeStr=Inherit: Same as accumulator  outputMin=[]  outputMax=[]  outputLastDataTypeStr=Inherit: Same as accumulator
      settings: SourceProductName=DSP System Toolbox
  Gain1 : Gain
  Gain2 : Gain  Gain=5
  Gain3 : Gain  Commented=on  Gain=10
  Gain4 : Gain  Gain=0.1
  PMApprox : Scope
  Product : Product
  Scope{,1..2,4} (4 alike) : Scope
  Zero-Order Hold : ZeroOrderHold  SampleTime=-1
  Zero-Order Hold3 : ZeroOrderHold  SampleTime=-1
  swY : Subsystem
  J1 : Outport
  ISE : Outport  Port=2
  OV : Outport  Port=3
  Ts : Outport  Port=4
  PM : Outport  Port=5
  wires:
  Cumulative Sum/1 -> Gain4/1, ISE/1, Scope2/1
  Zero-Order Hold3/1 -> Cumulative Sum/2
  e/1 -> Product/2, Product/1
  Zero-Order Hold/1 -> Cumulative Sum/1
  r/1 -> Zero-Order Hold3/1, Cost function/4(r)
  swY/1(O) -> Cost function/1(y)
  Clock/1 -> Cost function/2(time)
  Product/1 -> Zero-Order Hold/1
  Constant/1 -> Cost function/3(epsilon)
  y/1 -> Scope4/1, Cost function/6(yTotal), swY/1(I)
  Add4/1 -> J1/1
  Gain2/1 -> Add4/3
  period/1 -> Cost function/5(period)
  Constant1/1 -> Cost function/7(samplingTime)
  Gain1/1 -> Add4/2
  refAmplitude/1 -> Cost function/8(refAmplitude)
  Gain3/1 -> Add4/4
  Cost function/1(tsf) -> Gain1/1, Scope/1, Ts/1
  Cost function/2(ovf) -> Gain2/1, Scope1/1, OV/1
  Gain4/1 -> Add4/1

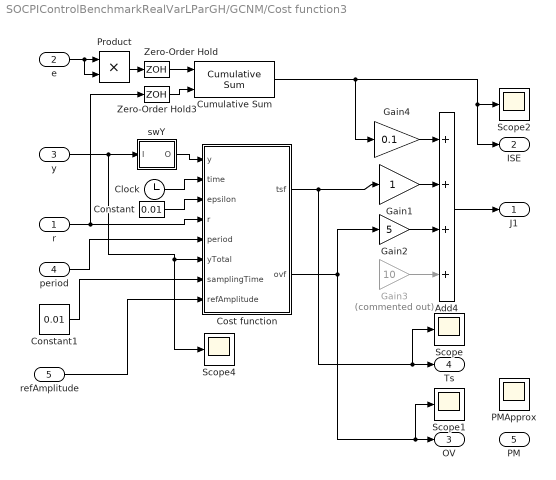
== system SOCPIControlBenchmarkRealVarLParGH/GCNM/Cost function3 ==
  r : Inport
  e : Inport  Port=2
  y : Inport  Port=3
  period : Inport  Port=4
  refAmplitude : Inport  Port=5
  Add4 : Sum  Inputs=++++
  Clock : Clock
  Constant : Constant  Value=0.01
  Constant1 : Constant  Value=0.01
  Cost function : MATLAB Function  TreatAsAtomicUnit=on
  Cumulative Sum : dspmathops/Cumulative Sum  dim=Channels (running sum)  InputProcessing=Columns as channels (frame based)  reset_popup=Falling edge  roundingMode=Floor  overflowMode=off  outputDataTypeStr=Inherit: Same as accumulator  outputMin=[]  outputMax=[]  outputLastDataTypeStr=Inherit: Same as accumulator
      settings: SourceProductName=DSP System Toolbox
  Gain1 : Gain
  Gain2 : Gain  Gain=5
  Gain3 : Gain  Commented=on  Gain=10
  Gain4 : Gain  Gain=0.1
  PMApprox : Scope
  Product : Product
  Scope{,1..2,4} (4 alike) : Scope
  Zero-Order Hold : ZeroOrderHold  SampleTime=-1
  Zero-Order Hold3 : ZeroOrderHold  SampleTime=-1
  swY : Subsystem
  J1 : Outport
  ISE : Outport  Port=2
  OV : Outport  Port=3
  Ts : Outport  Port=4
  PM : Outport  Port=5
  wires:
  Gain4/1 -> Add4/1
  Cost function/2(ovf) -> OV/1, Scope1/1, Gain2/1
  Cost function/1(tsf) -> Ts/1, Scope/1, Gain1/1
  Gain3/1 -> Add4/4
  refAmplitude/1 -> Cost function/8(refAmplitude)
  Gain1/1 -> Add4/2
  Constant1/1 -> Cost function/7(samplingTime)
  period/1 -> Cost function/5(period)
  Gain2/1 -> Add4/3
  Add4/1 -> J1/1
  y/1 -> swY/1(I), Cost function/6(yTotal), Scope4/1
  Constant/1 -> Cost function/3(epsilon)
  Product/1 -> Zero-Order Hold/1
  Clock/1 -> Cost function/2(time)
  swY/1(O) -> Cost function/1(y)
  r/1 -> Cost function/4(r), Zero-Order Hold3/1
  Zero-Order Hold/1 -> Cumulative Sum/1
  e/1 -> Product/1, Product/2
  Zero-Order Hold3/1 -> Cumulative Sum/2
  Cumulative Sum/1 -> Scope2/1, ISE/1, Gain4/1

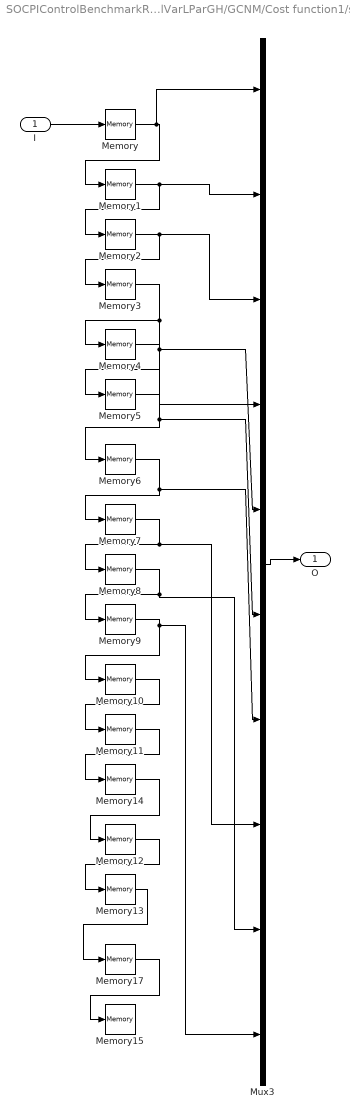
== system SOCPIControlBenchmarkRealVarLParGH/GCNM/Cost function1/swY ==
  I : Inport
  Memory{,1..15,17} (17 alike) : Memory
  Mux3 : Mux  Inputs=10
  O : Outport
  wires:
  Memory17/1 -> Memory15/1
  Memory7/1 -> Mux3/8, Memory8/1
  Memory/1 -> Mux3/1, Memory1/1
  Memory8/1 -> Mux3/9, Memory9/1
  I/1 -> Memory/1
  Memory2/1 -> Mux3/3, Memory3/1
  Memory10/1 -> Memory11/1
  Memory1/1 -> Mux3/2, Memory2/1
  Memory6/1 -> Mux3/7, Memory7/1
  Memory3/1 -> Mux3/4, Memory4/1
  Memory9/1 -> Mux3/10, Memory10/1
  Mux3/1 -> O/1
  Memory4/1 -> Mux3/5, Memory5/1
  Memory5/1 -> Mux3/6, Memory6/1
  Memory13/1 -> Memory17/1
  Memory12/1 -> Memory13/1
  Memory14/1 -> Memory12/1
  Memory11/1 -> Memory14/1

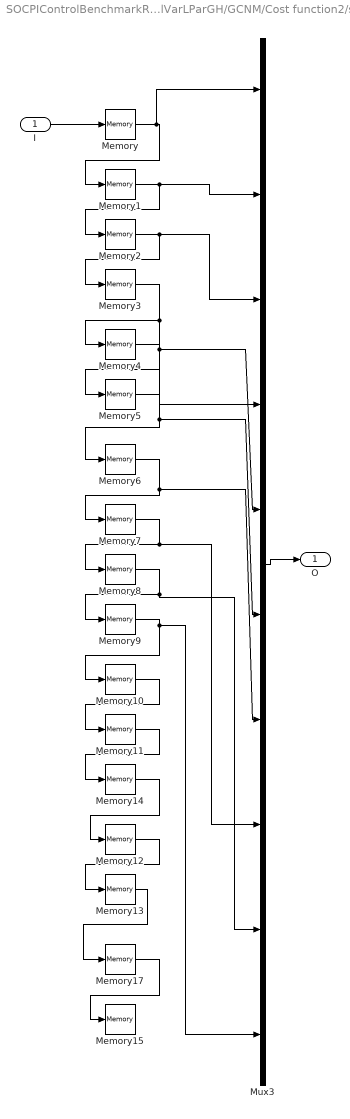
== system SOCPIControlBenchmarkRealVarLParGH/GCNM/Cost function2/swY ==
  I : Inport
  Memory{,1..15,17} (17 alike) : Memory
  Mux3 : Mux  Inputs=10
  O : Outport
  wires:
  Memory11/1 -> Memory14/1
  Memory14/1 -> Memory12/1
  Memory12/1 -> Memory13/1
  Memory13/1 -> Memory17/1
  Memory5/1 -> Memory6/1, Mux3/6
  Memory4/1 -> Memory5/1, Mux3/5
  Mux3/1 -> O/1
  Memory9/1 -> Memory10/1, Mux3/10
  Memory3/1 -> Memory4/1, Mux3/4
  Memory6/1 -> Memory7/1, Mux3/7
  Memory1/1 -> Memory2/1, Mux3/2
  Memory10/1 -> Memory11/1
  Memory2/1 -> Memory3/1, Mux3/3
  I/1 -> Memory/1
  Memory8/1 -> Memory9/1, Mux3/9
  Memory/1 -> Memory1/1, Mux3/1
  Memory7/1 -> Memory8/1, Mux3/8
  Memory17/1 -> Memory15/1

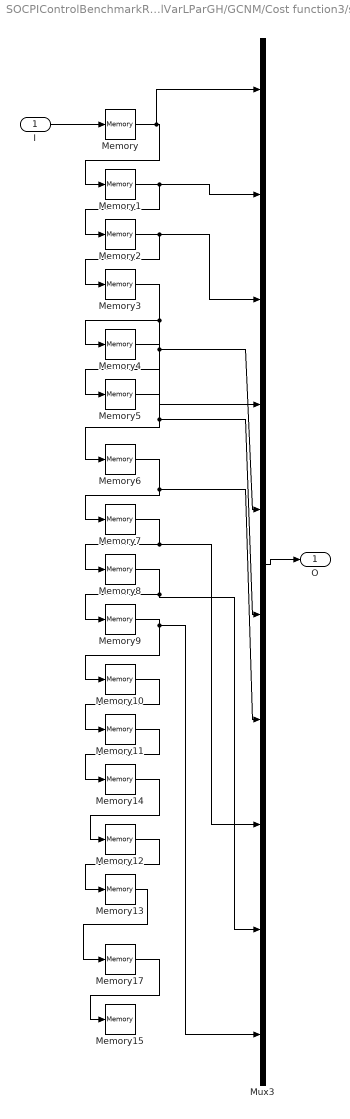
== system SOCPIControlBenchmarkRealVarLParGH/GCNM/Cost function3/swY ==
  I : Inport
  Memory{,1..15,17} (17 alike) : Memory
  Mux3 : Mux  Inputs=10
  O : Outport
  wires:
  Memory17/1 -> Memory15/1
  Memory7/1 -> Mux3/8, Memory8/1
  Memory/1 -> Mux3/1, Memory1/1
  Memory8/1 -> Mux3/9, Memory9/1
  I/1 -> Memory/1
  Memory2/1 -> Mux3/3, Memory3/1
  Memory10/1 -> Memory11/1
  Memory1/1 -> Mux3/2, Memory2/1
  Memory6/1 -> Mux3/7, Memory7/1
  Memory3/1 -> Mux3/4, Memory4/1
  Memory9/1 -> Mux3/10, Memory10/1
  Mux3/1 -> O/1
  Memory4/1 -> Mux3/5, Memory5/1
  Memory5/1 -> Mux3/6, Memory6/1
  Memory13/1 -> Memory17/1
  Memory12/1 -> Memory13/1
  Memory14/1 -> Memory12/1
  Memory11/1 -> Memory14/1

== matlab function SOCPIControlBenchmarkRealVarLParGH/Delay measurement ==
  data: u input; y output
function y = FOPDTDelayCalculation(u)

y = u;
